simulink model "CrustCrawlerSimulink"  (R2020b)
settings: Solver=VariableStepAuto  StartTime=0.0  StopTime=50  RelTol=1e-3
model workspace: external: MATLAB File C:\Users\soren\Documents\MATLAB\FinalAss_DataFile4.m (data not in the file)
undefined symbols (not defined in the file or in its folder): smiData, X, Y, Z
libraries: sm_lib x109, nesl_utility x16, simulink_extras x8
(part 3 of 3)

== matlab function CrustCrawlerSimulink/ Dynamics ==
  data: pos input; tau output; vel input; acc input
function tau = tauFunction(pos, vel, acc)

theta1 = pos(1)*pi/180; 
theta2 = pos(2)*pi/180;
theta3 = pos(3)*pi/180; 
theta4 = pos(4)*pi/180;

d_theta1 = vel(1)*pi/180; 
d_theta2 = vel(2)*pi/180; 
d_theta3 = vel(3)*pi/180; 
d_theta4 = vel(4)*pi/180;
%d_theta1 = 0; 
%d_theta2 = 0; 
%d_theta3 = 0;
%d_theta4 = 0;

dd_theta1 = acc(1)*pi/180; 
dd_theta2 = acc(2)*pi/180; 
dd_theta3 = acc(3)*pi/180; 
dd_theta4 = acc(4)*pi/180; 

ddd_theta1 = acc(1);
ddd_theta2 = acc(2);
ddd_theta3 = acc(3);
ddd_theta4 = acc(4);

%dd_theta1 = 0; 
%dd_theta2 = 0; 
%dd_theta3 = 0;
%dd_theta4 = 0;


%EOMFinal = [7.1746481373430634031294954664444e-43*dd_theta1*cos(theta3 + theta4) - dd_theta2*(0.00000050232007693581192964517441517593*cos(theta2 + theta3 - 0.0077990904512115243584117433454218) - 0.0000010273773424386293652240408631951*cos(theta2 - 0.16067188362009602389244175119891)) - 3.5873240686715317015647477332222e-43*dd_theta1*cos(2.0*theta2 + 2.0*theta3 + theta4) - 7.1746481373430634031294954664444e-43*dd_theta1*cos(2*theta2 + 2*theta3) - dd_theta3*(0.00000050232007693581192964517441517593*cos(theta2 + theta3 - 0.0077990904512115243584117433454218) + 0.0000044751091119323566162786748072789*cos(theta2 + 0.011561986867147647360931077407364)) - 1.1210387714598536567389836666319e-44*dd_theta1*sin(2*theta2 + 2*theta3) - 0.0000044751091119323566162786748072789*dd_theta4*cos(theta2 + 0.011561986867147647360931077407364) - 0.0000010141447399999987712512306003987*d_theta2^2*sin(theta2) - 7.1746481373430634031294954664444e-43*dd_theta1*cos(2.0*theta2 + theta3 + theta4) + 3.5032461608120426773093239582248e-46*dd_theta2*cos(theta2) + 3.5873240686715317015647477332222e-43*dd_theta1*cos(theta4) + 1.4012984643248170709237295832899e-45*dd_theta3*cos(theta2) + 1.4012984643248170709237295832899e-45*dd_theta4*cos(theta2) + 4.379057701015053346636654947781e-47*dd_theta2*sin(theta2) - 0.0000000039176000000000000441085419260862*d_theta2^2*cos(theta2 + theta3) - 0.0000000039176000000000000441085419260862*d_theta3^2*cos(theta2 + theta3) + 0.00000050230480000000001604358518866172*d_theta2^2*sin(theta2 + theta3) + 0.00000050230480000000001604358518866172*d_theta3^2*sin(theta2 + theta3) - dd_theta1*(0.0026664215522818742773049238562024*cos(2.0*theta2 + theta3 + theta4 - 0.37167538659543453160431952857526) - 0.0026664215522818742773049238562024*cos(theta3 + theta4 - 0.37167538659543453160431952857526) + 0.011645192380542018999411409110892*cos(2.0*theta2 - 0.0049035858392241764753990490096684) + 0.0025875830098561777741379419949728*cos(2.0*theta2 + 2.0*theta3 - 0.0083023869461122679538775545739355) + 0.0004562011636*cos(2.0*theta2 + 2.0*theta3 + 2.0*theta4 - 0.74335077319086906320863905715051) - 0.0017816544008428887216537445766443*cos(theta4 - 0.37167538659543453160431952857526) - 0.0082519140353150068428276331824979*cos(theta3 - 0.0071552010307614737572427569454836) + 0.0017816544008428887216537445766443*cos(2.0*theta2 + 2.0*theta3 + theta4 - 0.37167538659543453160431952857526) + 0.0082519140353150068428276331824979*cos(2.0*theta2 + theta3 - 0.0071552010307614737572427569454836) - 0.014986765501069999986146902997142) + 0.00000016436133999999999751962027460389*d_theta2^2*cos(theta2) + 0.0000590436*d_theta1*d_theta3*cos(theta3) + 0.000000051739999999999998759810137301946*d_theta2*d_theta3*cos(theta2) + 0.000000051739999999999998759810137301946*d_theta2*d_theta4*cos(theta2) + 0.00064705578*d_theta1*d_theta4*cos(theta4) - 0.0082517028*d_theta1*d_theta3*sin(theta3) + 0.0000044748100000000006143743846998007*d_theta2*d_theta3*sin(theta2) + 0.0000044748100000000006143743846998007*d_theta2*d_theta4*sin(theta2) - 0.00166000338*d_theta1*d_theta4*sin(theta4) - 0.0006174760872*d_theta1*d_theta2*cos(2*theta2 + 2*theta3 + 2*theta4) - 0.0006174760872*d_theta1*d_theta3*cos(2*theta2 + 2*theta3 + 2*theta4) - 0.0006174760872*d_theta1*d_theta4*cos(2*theta2 + 2*theta3 + 2*theta4) - 0.0001180872*d_theta1*d_theta2*cos(2.0*theta2 + theta3) - 0.0000590436*d_theta1*d_theta3*cos(2.0*theta2 + theta3) + 0.000671715184*d_theta1*d_theta2*sin(2*theta2 + 2*theta3 + 2*theta4) + 0.000671715184*d_theta1*d_theta3*sin(2*theta2 + 2*theta3 + 2*theta4) + 0.000671715184*d_theta1*d_theta4*sin(2*theta2 + 2*theta3 + 2*theta4) + 0.0165034056*d_theta1*d_theta2*sin(2.0*theta2 + theta3) + 0.0082517028*d_theta1*d_theta3*sin(2.0*theta2 + theta3) - 0.00129411156*d_theta1*d_theta2*cos(2.0*theta2 + 2.0*theta3 + theta4) - 0.00129411156*d_theta1*d_theta3*cos(2.0*theta2 + 2.0*theta3 + theta4) - 0.00064705578*d_theta1*d_theta4*cos(2.0*theta2 + 2.0*theta3 + theta4) - 0.000042965737199999999183934694391151*d_theta1*d_theta2*cos(2*theta2 + 2*theta3) - 0.000042965737199999999183934694391151*d_theta1*d_theta3*cos(2*theta2 + 2*theta3) + 0.00332000676*d_theta1*d_theta2*sin(2.0*theta2 + 2.0*theta3 + theta4) + 0.00332000676*d_theta1*d_theta3*sin(2.0*theta2 + 2.0*theta3 + theta4) + 0.00166000338*d_theta1*d_theta4*sin(2.0*theta2 + 2.0*theta3 + theta4) - 0.0001142059432200000029456992400867*d_theta1*d_theta2*cos(2.0*theta2) + 0.005174987659599999988342437307054*d_theta1*d_theta2*sin(2*theta2 + 2*theta3) + 0.005174987659599999988342437307054*d_theta1*d_theta3*sin(2*theta2 + 2*theta3) + 0.023290104751199999957260424787719*d_theta1*d_theta2*sin(2.0*theta2) - 0.0000000078352000000000000882170838521724*d_theta2*d_theta3*cos(theta2 + theta3) + 0.0009683828*d_theta1*d_theta3*cos(theta3 + theta4) + 0.0009683828*d_theta1*d_theta4*cos(theta3 + theta4) + 0.0000010046096000000000320871703773234*d_theta2*d_theta3*sin(theta2 + theta3) - 0.0024843588*d_theta1*d_theta3*sin(theta3 + theta4) - 0.0024843588*d_theta1*d_theta4*sin(theta3 + theta4) - 0.0019367656*d_theta1*d_theta2*cos(2.0*theta2 + theta3 + theta4) - 0.0009683828*d_theta1*d_theta3*cos(2.0*theta2 + theta3 + theta4) - 0.0009683828*d_theta1*d_theta4*cos(2.0*theta2 + theta3 + theta4) + 0.0049687176*d_theta1*d_theta2*sin(2.0*theta2 + theta3 + theta4) + 0.0024843588*d_theta1*d_theta3*sin(2.0*theta2 + theta3 + theta4) + 0.0024843588*d_theta1*d_theta4*sin(2.0*theta2 + theta3 + theta4)
%                                                                                                                                                                                                                                                                                                                                                                                                                                                                                                                                                                                                                                                                                                                                                                                                                                                                                                                                                                                                                                                                                                                                                                                                                                                                                                                                9.2014687540397668648947902489241e-41*cos(theta2 + theta3 + 1.5083775167989392707573425786543) + 0.36833543557633348725712435387331*cos(theta2 + theta3 + 1.5636411257641351454740789346943) + 0.11901936201549093365061069212685*cos(theta2 + theta3 + theta4 + 1.1991209401994620876270021630645) - 2.2958874039497802890014385492622e-41*cos(theta2 + theta3 + theta4 + 1.1991209401994620876270021630645) + 1.0545256522014907407374294396952*cos(theta2 + 1.5686157793635218984342744391719) + 1.7864873861984227873792443711446e-40*cos(theta2) + dd_theta3*(0.0026664215522818742773049238562024*cos(theta3 + theta4 - 0.37167538659543453160431952857526) + 0.0035633088016857774433074891532886*cos(theta4 - 0.37167538659543453160431952857526) + 0.0082519140353150068428276331824979*cos(theta3 - 0.0071552010307614737572427569454836) + 0.0062267178731999999919430743178239) - 0.0082517028*d_theta3^2*sin(theta3) - 0.00166000338*d_theta4^2*sin(theta4) + dd_theta2*(0.0053328431045637485546098477124047*cos(theta3 + theta4 - 0.37167538659543453160431952857526) + 0.0035633088016857774433074891532886*cos(theta4 - 0.37167538659543453160431952857526) + 0.016503828070630013685655266364996*cos(theta3 - 0.0071552010307614737572427569454836) + 0.027315394567419999995747989034456) - dd_theta1*(0.00000050232007693581192964517441517593*cos(theta2 + theta3 - 0.0077990904512115243584117433454218) - 0.0000010273773424386293652240408631951*cos(theta2 - 0.16067188362009602389244175119891)) + 0.0003087380436*d_theta1^2*cos(2*theta2 + 2*theta3 + 2*theta4) + 0.0000590436*d_theta1^2*cos(2.0*theta2 + theta3) + 1.4349296274686126806258990932889e-42*dd_theta2*cos(theta3 + theta4) + 7.1746481373430634031294954664444e-43*dd_theta3*cos(theta3 + theta4) + 7.1746481373430634031294954664444e-43*dd_theta4*cos(theta3 + theta4) - 0.000335857592*d_theta1^2*sin(2*theta2 + 2*theta3 + 2*theta4) - 0.0082517028*d_theta1^2*sin(2.0*theta2 + theta3) + 0.00064705578*d_theta1^2*cos(2.0*theta2 + 2.0*theta3 + theta4) + 0.000021482868599999999591967347195576*d_theta1^2*cos(2*theta2 + 2*theta3) - 0.00166000338*d_theta1^2*sin(2.0*theta2 + 2.0*theta3 + theta4) + dd_theta4*(0.0026664215522818742773049238562024*cos(theta3 + theta4 - 0.37167538659543453160431952857526) + 0.0017816544008428887216537445766443*cos(theta4 - 0.37167538659543453160431952857526) + 0.0010318093272000000038049147166319) + 0.000057102971610000001472849620043348*d_theta1^2*cos(2.0*theta2) + 3.5032461608120426773093239582248e-46*dd_theta1*cos(theta2) + 7.1746481373430634031294954664444e-43*dd_theta2*cos(theta4) + 7.1746481373430634031294954664444e-43*dd_theta3*cos(theta4) + 3.5873240686715317015647477332222e-43*dd_theta4*cos(theta4) - 0.002587493829799999994171218653527*d_theta1^2*sin(2*theta2 + 2*theta3) - 0.01164505237559999997863021239386*d_theta1^2*sin(2.0*theta2) + 4.379057701015053346636654947781e-47*dd_theta1*sin(theta2) + 0.0009683828*d_theta3^2*cos(theta3 + theta4) + 0.0009683828*d_theta4^2*cos(theta3 + theta4) - 0.0024843588*d_theta3^2*sin(theta3 + theta4) - 0.0024843588*d_theta4^2*sin(theta3 + theta4) + 0.0009683828*d_theta1^2*cos(2.0*theta2 + theta3 + theta4) - 0.0024843588*d_theta1^2*sin(2.0*theta2 + theta3 + theta4) + 0.0000590436*d_theta3^2*cos(theta3) + 0.00064705578*d_theta4^2*cos(theta4) - 0.000000051739999999999998759810137301946*d_theta1*d_theta3*cos(theta2) - 0.000000051739999999999998759810137301946*d_theta1*d_theta4*cos(theta2) + 0.0001180872*d_theta2*d_theta3*cos(theta3) + 0.00129411156*d_theta2*d_theta4*cos(theta4) + 0.00129411156*d_theta3*d_theta4*cos(theta4) - 0.0000044748100000000006143743846998007*d_theta1*d_theta3*sin(theta2) - 0.0000044748100000000006143743846998007*d_theta1*d_theta4*sin(theta2) - 0.0165034056*d_theta2*d_theta3*sin(theta3) - 0.00332000676*d_theta2*d_theta4*sin(theta4) - 0.00332000676*d_theta3*d_theta4*sin(theta4) + 0.0019367656*d_theta2*d_theta3*cos(theta3 + theta4) + 0.0019367656*d_theta2*d_theta4*cos(theta3 + theta4) + 0.0019367656*d_theta3*d_theta4*cos(theta3 + theta4) - 0.0049687176*d_theta2*d_theta3*sin(theta3 + theta4) - 0.0049687176*d_theta2*d_theta4*sin(theta3 + theta4) - 0.0049687176*d_theta3*d_theta4*sin(theta3 + theta4)
%                                                                                                                                                                                                                                                                                                                                                                                                                                                                                                                                                                                                                                                                                                                                                                                                                                                                                                                                                                                                                                                                                                                                                                                                                                                                                                                                                                                                                                                                                                                                                                                                                                                                                                                                                                                                                                                                                                                                                                                                                                                                                                                                                                                                                                                                                                                                                                                                                                                                                                                                                                                                                    9.2014687540397668648947902489241e-41*cos(theta2 + theta3 + 1.5083775167989392707573425786543) + 0.36833543557633348725712435387331*cos(theta2 + theta3 + 1.5636411257641351454740789346943) + 0.11901936201549093365061069212685*cos(theta2 + theta3 + theta4 + 1.1991209401994620876270021630645) - 2.2958874039497802890014385492622e-41*cos(theta2 + theta3 + theta4 + 1.1991209401994620876270021630645) + dd_theta2*(0.0026664215522818742773049238562024*cos(theta3 + theta4 - 0.37167538659543453160431952857526) + 0.0035633088016857774433074891532886*cos(theta4 - 0.37167538659543453160431952857526) + 0.0082519140353150068428276331824979*cos(theta3 - 0.0071552010307614737572427569454836) + 0.0062267178731999999919430743178239) + 0.0041258514*d_theta1^2*sin(theta3) + 0.0082517028*d_theta2^2*sin(theta3) - 0.00166000338*d_theta4^2*sin(theta4) - dd_theta1*(0.00000050232007693581192964517441517593*cos(theta2 + theta3 - 0.0077990904512115243584117433454218) + 0.0000044751091119323566162786748072789*cos(theta2 + 0.011561986867147647360931077407364)) + 0.0003087380436*d_theta1^2*cos(2*theta2 + 2*theta3 + 2*theta4) + 0.0000295218*d_theta1^2*cos(2.0*theta2 + theta3) + 7.1746481373430634031294954664444e-43*dd_theta2*cos(theta3 + theta4) - 0.000335857592*d_theta1^2*sin(2*theta2 + 2*theta3 + 2*theta4) - 0.0041258514*d_theta1^2*sin(2.0*theta2 + theta3) + 0.00064705578*d_theta1^2*cos(2.0*theta2 + 2.0*theta3 + theta4) + 0.000021482868599999999591967347195576*d_theta1^2*cos(2*theta2 + 2*theta3) - 0.00166000338*d_theta1^2*sin(2.0*theta2 + 2.0*theta3 + theta4) + 1.4012984643248170709237295832899e-45*dd_theta1*cos(theta2) + 7.1746481373430634031294954664444e-43*dd_theta2*cos(theta4) + 7.1746481373430634031294954664444e-43*dd_theta3*cos(theta4) + 3.5873240686715317015647477332222e-43*dd_theta4*cos(theta4) - 0.002587493829799999994171218653527*d_theta1^2*sin(2*theta2 + 2*theta3) - 0.0004841914*d_theta1^2*cos(theta3 + theta4) - 0.0009683828*d_theta2^2*cos(theta3 + theta4) + dd_theta4*(0.0017816544008428887216537445766443*cos(theta4 - 0.37167538659543453160431952857526) + 0.0010318093272000000038049147166319) + 0.0012421794*d_theta1^2*sin(theta3 + theta4) + 0.0024843588*d_theta2^2*sin(theta3 + theta4) + 0.0004841914*d_theta1^2*cos(2.0*theta2 + theta3 + theta4) - 0.0012421794*d_theta1^2*sin(2.0*theta2 + theta3 + theta4) + dd_theta3*(0.0035633088016857774433074891532886*cos(theta4 - 0.37167538659543453160431952857526) + 0.0062267178731999999919430743178239) - 0.0000295218*d_theta1^2*cos(theta3) - 0.0000590436*d_theta2^2*cos(theta3) + 0.00064705578*d_theta4^2*cos(theta4) + 0.000000051739999999999998759810137301946*d_theta1*d_theta2*cos(theta2) + 0.00129411156*d_theta2*d_theta4*cos(theta4) + 0.00129411156*d_theta3*d_theta4*cos(theta4) + 0.0000044748100000000006143743846998007*d_theta1*d_theta2*sin(theta2) - 0.00332000676*d_theta2*d_theta4*sin(theta4) - 0.00332000676*d_theta3*d_theta4*sin(theta4)
%                                                                                                                                                                                                                                                                                                                                                                                                                                                                                                                                                                                                                                                                                                                                                                                                                                                                                                                                                                                                                                                                                                                                                                                                                                                                                                                                                                                                                                                                                                                                                                                                                                                                                                                                                                                                                                                                                                                                                                                                                                                                                                                                                                                                                                                                                                                                                                                                                                                                                                                                                                                                                                                                                                                                                                                                                                                                                                                                                                                                                                                                                                                                                                                                                                                                                                                                                                                                                                                                                                                                   0.0010318093272000000038049147166319*dd_theta4 + 0.11901936201549093365061069212685*cos(theta2 + theta3 + theta4 + 1.1991209401994620876270021630645) - 2.2958874039497802890014385492622e-41*cos(theta2 + theta3 + theta4 + 1.1991209401994620876270021630645) + 0.00083000169*d_theta1^2*sin(theta4) + 0.00166000338*d_theta2^2*sin(theta4) + 0.00166000338*d_theta3^2*sin(theta4) - 0.0000044751091119323566162786748072789*dd_theta1*cos(theta2 + 0.011561986867147647360931077407364) + 0.0003087380436*d_theta1^2*cos(2*theta2 + 2*theta3 + 2*theta4) + 7.1746481373430634031294954664444e-43*dd_theta2*cos(theta3 + theta4) - 0.000335857592*d_theta1^2*sin(2*theta2 + 2*theta3 + 2*theta4) + 0.00032352789*d_theta1^2*cos(2.0*theta2 + 2.0*theta3 + theta4) - 0.00083000169*d_theta1^2*sin(2.0*theta2 + 2.0*theta3 + theta4) + dd_theta2*(0.0026664215522818742773049238562024*cos(theta3 + theta4 - 0.37167538659543453160431952857526) + 0.0017816544008428887216537445766443*cos(theta4 - 0.37167538659543453160431952857526) + 0.0010318093272000000038049147166319) + 1.4012984643248170709237295832899e-45*dd_theta1*cos(theta2) + 3.5873240686715317015647477332222e-43*dd_theta2*cos(theta4) + 3.5873240686715317015647477332222e-43*dd_theta3*cos(theta4) - 0.0004841914*d_theta1^2*cos(theta3 + theta4) - 0.0009683828*d_theta2^2*cos(theta3 + theta4) + dd_theta3*(0.0017816544008428887216537445766443*cos(theta4 - 0.37167538659543453160431952857526) + 0.0010318093272000000038049147166319) + 0.0012421794*d_theta1^2*sin(theta3 + theta4) + 0.0024843588*d_theta2^2*sin(theta3 + theta4) + 0.0004841914*d_theta1^2*cos(2.0*theta2 + theta3 + theta4) - 0.0012421794*d_theta1^2*sin(2.0*theta2 + theta3 + theta4) - 0.00032352789*d_theta1^2*cos(theta4) - 0.00064705578*d_theta2^2*cos(theta4) - 0.00064705578*d_theta3^2*cos(theta4) + 0.000000051739999999999998759810137301946*d_theta1*d_theta2*cos(theta2) - 0.00129411156*d_theta2*d_theta3*cos(theta4) + 0.0000044748100000000006143743846998007*d_theta1*d_theta2*sin(theta2) + 0.00332000676*d_theta2*d_theta3*sin(theta4)];
%                                                                                                                                                                                                                                                                                                                                                                                                                                                                                                                                                                                                                                                                                                                                                                                                                                                                                                                                                                                                                                                                                                                                                                                                                                                                                                                                                                                                                                                                                                                                                                                                                                                                                                                                                                                                                                                                                                                                                                                                                                                                                                                                                                                                                                                                                                                                                                                                                                                                                                                                                                                                                                                                                                                                                                                                                                                                                                                                                                                                                                                                                                                                                                                                                                                                                                                                                                                                                                                                                                                               
M11 = 0.0027*cos(theta3 + theta4 - 0.3717) - 0.0027*cos(2.0*theta2 + theta3 + theta4 - 0.3717) - 0.0116*cos(2.0*theta2 - 0.0049) - 0.0026*cos(2.0*theta2 + 2.0*theta3 - 0.0083) - 0.0005*cos(2.0*theta2 + 2.0*theta3 + 2.0*theta4 - 0.7434) + 0.0018*cos(theta4 - 0.3717) + 0.0083*cos(theta3 - 0.0072) - 0.0018*cos(2.0*theta2 + 2.0*theta3 + theta4 - 0.3717) - 0.0083*cos(2.0*theta2 + theta3 - 0.0072) + 0.0150;
M22 = 0.0053*cos(theta3 + theta4 - 0.3717) + 0.0036*cos(theta4 - 0.3717) + 0.0165*cos(theta3 - 0.0072) + 0.0273;
M33 = 0.0036*cos(theta4 - 0.3717) + 0.0062;
M44 = 0.0010;                                                                                                                                                                                                                                                                                                                                                                                                                                                                                                                                                                                                                                                                                                                                                                                                                                                                                                                                                                                                                                                                                                                                                                                                                                                                                                                                                                                                                                                                                                                                                                                                                                                                                                                                                                                                                                                                                                                                                                                                                                                                                                                                                                                                                                                                                                                                                                                                                                                                                                                                                                                                                                                                                                                                                                                                                                                                                                                                                                                                                                                                                                                                                                                                                                                                                                                                                                                                                                                                                                                               

CG1 = 0.0006*d_theta1*d_theta4*cos(theta4) - 0.0083*d_theta1*d_theta3*sin(theta3) - 0.0017*d_theta1*d_theta4*sin(theta4) - 0.0006*d_theta1*d_theta2*cos(2*theta2 + 2*theta3 + 2*theta4) - 0.0006*d_theta1*d_theta3*cos(2*theta2 + 2*theta3 + 2*theta4) - 0.0006*d_theta1*d_theta4*cos(2*theta2 + 2*theta3 + 2*theta4) - 0.0001*d_theta1*d_theta2*cos(2.0*theta2 + theta3) + 0.0007*d_theta1*d_theta2*sin(2*theta2 + 2*theta3 + 2*theta4) + 0.0007*d_theta1*d_theta3*sin(2*theta2 + 2*theta3 + 2*theta4) + 0.0007*d_theta1*d_theta4*sin(2*theta2 + 2*theta3 + 2*theta4) + 0.0165*d_theta1*d_theta2*sin(2.0*theta2 + theta3) + 0.0083*d_theta1*d_theta3*sin(2.0*theta2 + theta3) - 0.0013*d_theta1*d_theta2*cos(2.0*theta2 + 2.0*theta3 + theta4) - 0.0013*d_theta1*d_theta3*cos(2.0*theta2 + 2.0*theta3 + theta4) - 0.0006*d_theta1*d_theta4*cos(2.0*theta2 + 2.0*theta3 + theta4) + 0.0033*d_theta1*d_theta2*sin(2.0*theta2 + 2.0*theta3 + theta4) + 0.0033*d_theta1*d_theta3*sin(2.0*theta2 + 2.0*theta3 + theta4) + 0.0017*d_theta1*d_theta4*sin(2.0*theta2 + 2.0*theta3 + theta4) - 0.0001*d_theta1*d_theta2*cos(2.0*theta2) + 0.0052*d_theta1*d_theta2*sin(2*theta2 + 2*theta3) + 0.0052*d_theta1*d_theta3*sin(2*theta2 + 2*theta3) + 0.0233*d_theta1*d_theta2*sin(2.0*theta2) + 0.0010*d_theta1*d_theta3*cos(theta3 + theta4) + 0.0010*d_theta1*d_theta4*cos(theta3 + theta4) - 0.0025*d_theta1*d_theta3*sin(theta3 + theta4) - 0.0025*d_theta1*d_theta4*sin(theta3 + theta4) - 0.0020*d_theta1*d_theta2*cos(2.0*theta2 + theta3 + theta4) - 0.0010*d_theta1*d_theta3*cos(2.0*theta2 + theta3 + theta4) - 0.0010*d_theta1*d_theta4*cos(2.0*theta2 + theta3 + theta4) + 0.0050*d_theta1*d_theta2*sin(2.0*theta2 + theta3 + theta4) + 0.0025*d_theta1*d_theta3*sin(2.0*theta2 + theta3 + theta4) + 0.0025*d_theta1*d_theta4*sin(2.0*theta2 + theta3 + theta4);
CG2 = 0.3683*cos(theta2 + theta3 + 1.5636) + 0.1190*cos(theta2 + theta3 + theta4 + 1.1991) + 1.0545*cos(theta2 + 1.5686) - 0.0083*d_theta3^2*sin(theta3) - 0.0017*d_theta4^2*sin(theta4) + 0.0003*d_theta1^2*cos(2*theta2 + 2*theta3 + 2*theta4) + 0.0001*d_theta1^2*cos(2.0*theta2 + theta3) - 0.0003*d_theta1^2*sin(2*theta2 + 2*theta3 + 2*theta4) - 0.0083*d_theta1^2*sin(2.0*theta2 + theta3) + 0.0006*d_theta1^2*cos(2.0*theta2 + 2.0*theta3 + theta4) - 0.0017*d_theta1^2*sin(2.0*theta2 + 2.0*theta3 + theta4) + 0.0001*d_theta1^2*cos(2.0*theta2) - 0.0026*d_theta1^2*sin(2*theta2 + 2*theta3) - 0.0116*d_theta1^2*sin(2.0*theta2) + 0.0010*d_theta3^2*cos(theta3 + theta4) + 0.0010*d_theta4^2*cos(theta3 + theta4) - 0.0025*d_theta3^2*sin(theta3 + theta4) - 0.0025*d_theta4^2*sin(theta3 + theta4) + 0.0010*d_theta1^2*cos(2.0*theta2 + theta3 + theta4) - 0.0025*d_theta1^2*sin(2.0*theta2 + theta3 + theta4) + 0.0006*d_theta4^2*cos(theta4) + 0.0001*d_theta2*d_theta3*cos(theta3) + 0.0013*d_theta2*d_theta4*cos(theta4) + 0.0013*d_theta3*d_theta4*cos(theta4) - 0.0165*d_theta2*d_theta3*sin(theta3) - 0.0033*d_theta2*d_theta4*sin(theta4) - 0.0033*d_theta3*d_theta4*sin(theta4) + 0.0020*d_theta2*d_theta3*cos(theta3 + theta4) + 0.0020*d_theta2*d_theta4*cos(theta3 + theta4) + 0.0020*d_theta3*d_theta4*cos(theta3 + theta4) - 0.0050*d_theta2*d_theta3*sin(theta3 + theta4) - 0.0050*d_theta2*d_theta4*sin(theta3 + theta4) - 0.0050*d_theta3*d_theta4*sin(theta3 + theta4);
CG3 = 0.3683*cos(theta2 + theta3 + 1.5636) + 0.1190*cos(theta2 + theta3 + theta4 + 1.1991) + 0.0041*d_theta1^2*sin(theta3) + 0.0083*d_theta2^2*sin(theta3) - 0.0017*d_theta4^2*sin(theta4) + 0.0003*d_theta1^2*cos(2*theta2 + 2*theta3 + 2*theta4) - 0.0003*d_theta1^2*sin(2*theta2 + 2*theta3 + 2*theta4) - 0.0041*d_theta1^2*sin(2.0*theta2 + theta3) + 0.0006*d_theta1^2*cos(2.0*theta2 + 2.0*theta3 + theta4) - 0.0017*d_theta1^2*sin(2.0*theta2 + 2.0*theta3 + theta4) - 0.0026*d_theta1^2*sin(2*theta2 + 2*theta3) - 0.0005*d_theta1^2*cos(theta3 + theta4) - 0.0010*d_theta2^2*cos(theta3 + theta4) + 0.0012*d_theta1^2*sin(theta3 + theta4) + 0.0025*d_theta2^2*sin(theta3 + theta4) + 0.0005*d_theta1^2*cos(2.0*theta2 + theta3 + theta4) - 0.0012*d_theta1^2*sin(2.0*theta2 + theta3 + theta4) - 0.0001*d_theta2^2*cos(theta3) + 0.0006*d_theta4^2*cos(theta4) + 0.0013*d_theta2*d_theta4*cos(theta4) + 0.0013*d_theta3*d_theta4*cos(theta4) - 0.0033*d_theta2*d_theta4*sin(theta4) - 0.0033*d_theta3*d_theta4*sin(theta4);
CG4 = 0.1190*cos(theta2 + theta3 + theta4 + 1.1991) + 0.0008*d_theta1^2*sin(theta4) + 0.0017*d_theta2^2*sin(theta4) + 0.0017*d_theta3^2*sin(theta4) + 0.0003*d_theta1^2*cos(2*theta2 + 2*theta3 + 2*theta4) - 0.0003*d_theta1^2*sin(2*theta2 + 2*theta3 + 2*theta4) + 0.0003*d_theta1^2*cos(2.0*theta2 + 2.0*theta3 + theta4) - 0.0008*d_theta1^2*sin(2.0*theta2 + 2.0*theta3 + theta4) - 0.0005*d_theta1^2*cos(theta3 + theta4) - 0.0010*d_theta2^2*cos(theta3 + theta4) + 0.0012*d_theta1^2*sin(theta3 + theta4) + 0.0025*d_theta2^2*sin(theta3 + theta4) + 0.0005*d_theta1^2*cos(2.0*theta2 + theta3 + theta4) - 0.0012*d_theta1^2*sin(2.0*theta2 + theta3 + theta4) - 0.0003*d_theta1^2*cos(theta4) - 0.0006*d_theta2^2*cos(theta4) - 0.0006*d_theta3^2*cos(theta4) - 0.0013*d_theta2*d_theta3*cos(theta4) + 0.0033*d_theta2*d_theta3*sin(theta4);

%tau = [EOMFinal(1); EOMFinal(2); EOMFinal(3); EOMFinal(4)]
tau = [M11*ddd_theta1+CG1; M22*ddd_theta2+CG2; M33*ddd_theta3+CG3; M44*ddd_theta4+CG4]

== matlab function CrustCrawlerSimulink/MATLAB Function3 ==
  data: t1 input; Pos output; t2 input; t3 input; t4 input
%% Crustecrwler forward kinematics
function Pos  = ForwardKinFunction(t1, t2, t3, t4)
theta1 = t1*pi/180;
theta2 = t2*pi/180;
theta3 = t3*pi/180;
theta4 = t4*pi/180;
% Denne section udregner Matricen T04, med de vinkler vi selv s?tter ind
% t1, t2, t3 og t4 beskriver theta vinklerne i hver motor
%Vinklerne inds?ttes i denavit hartenberg parameterne for vores robot:
T01=TDH(0,0,0,theta1+90*pi/180)
T12=TDH(-90*pi/180,0,0,theta2-90*pi/180)
T23=TDH(0,220,0,theta3);
T34=TDH(0,147,0,theta4);
%Base to final joint
T04=T01*T12*T23*T34;
Pos=[T04(1,4); T04(2,4); T04(3,4)]
